simulink model "pt2_matlabfun"  (R2015b)
settings: Solver=ode45  StartTime=0.0  StopTime=20e-3  RelTol=1e-3
InitFcn:
  | pt2_data;
values from neighbouring files (symbols this model uses):
  P_D = 0.3    [pt2_data.m]
  P_k = 1    [pt2_data.m]
  P_T = 1e-3    (= 0.001)    [pt2_data.m]
  P_u_step = 2    [pt2_data.m]
  P_u_steptime = 1e-3    (= 0.001)    [pt2_data.m]
  P_v0 = 0    [pt2_data.m]
  P_x0 = 0    [pt2_data.m]
settings Model: Creator=traenkle  LastModifiedBy=ftraenkle
settings DataIOCC: SaveFormat=Array  InspectSignalLogs=on
settings DebuggingCC: UnderspecifiedInitializationDetection=Classic  MergeDetectMultiDrivingBlocksExec=none  SolverPrmCheckMsg=warning  MultiTaskDSMMsg=warning  MultiTaskCondExecSysMsg=none  StateNameClashWarn=warning
settings HardwareCC: ProdBitPerPointer=32  ProdLargestAtomicFloat=None  ProdIntDivRoundTo=Undefined  ProdEndianess=Unspecified  ProdWordSize=32  ProdHWDeviceType=32-bit Generic
settings GRTTargetCC: GeneratePreprocessorConditionals=Disable all
settings ConfigComp: CovModelRefEnable=Off

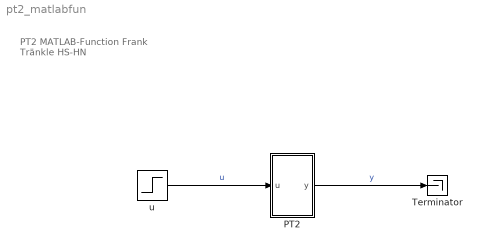
== system pt2_matlabfun ==
  note: PT2 MATLAB-Function
      | Frank Tränkle
      | HS-HN
  PT2 : Subsystem
  Terminator : Terminator
  u : Step  Time=P_u_steptime  After=P_u_step  SampleTime=0
  wires:
  u/1 -> PT2/1(u)  "u"
  PT2/1(y) -> Terminator/1  "y"

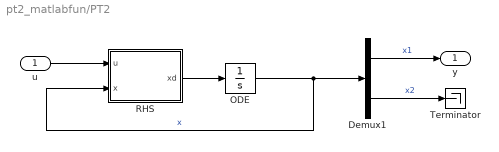
== system pt2_matlabfun/PT2 ==
  u : Inport
  Demux1 : Demux  Outputs=2
  ODE : Integrator  InitialCondition=[ P_x0 P_v0 ]
  RHS : MATLAB Function  TreatAsAtomicUnit=on
  Terminator : Terminator
  y : Outport
  wires:
  ODE/1 -> RHS/2(x), Demux1/1  "x"
  Demux1/1 -> y/1  "x1"
  Demux1/2 -> Terminator/1  "x2"
  RHS/1(xd) -> ODE/1
  u/1 -> RHS/1(u)

== matlab function pt2_matlabfun/PT2/RHS ==
  data: u input; xd output; x input; P_k parameter; P_T parameter; P_D parameter
function xd = f(u, x, P_k, P_T, P_D)
%#codegen
xd = [ x(2); ...
    (-x(1) - 2*P_D*P_T * x(2) + P_k * u) / (P_T * P_T) ];
end
